simulink model "dspace"  (R2021b)
settings: Solver=FixedStepDiscrete  StartTime=0.0  StopTime=Inf  FixedStep=1e-3  RelTol=1e-3
PostLoadFcn:
  | , if any(exist('dsrtsu_mdlpostloadfcn', 'file') ~= 0), dsrtsu_mdlpostloadfcn('Execute', bdroot); end,
undefined symbols (not defined in the file): ami, amk1_setpoints_1, amk2_setpoints_1, amk3_setpoints_1, amk4_setpoints_1, as, digital, ebs, indicator, mcu_set_dbu_indicator_points, mcu_set_ecu_indicator_points, res_ntm_node_control
libraries: rtican x63, rti1401lib_dio_type3 x4, simulink x4, simulink_extras x1
(part 6 of 16)

== system dspace/CAN RX/amk1_actual_values_2 ==
  amk1_actual_values_21 : rtican/RTICAN Receive (RX)   Reserved1=[]  Reserved2=[]  Reserved3=[]  Reserved4=[]  SfcnMessage=[]  Msg_Struct=[]  BoardTypeNo=[]  BoardNo=[]  ChannelNo=[]  Parameters=[]  DialogFcn=[]  UnitName=[]  Revision=[]  UnitValues=[]  DSProperties=struct('RTI',struct('Version',uint32(5),'BlockType',struct('isSLSource',uint8(1),'isSLSink',uint8(1),'isHWSource',uint8(0),'isHWSink',uint8(0),'isSetup',uint8(0),'isInline',uint8(1),'isNonInline',uint8(0),'isInterrupt',uint8(0),'isChannelwise',uint8(0)),'IOBoardType','RTICAN','UnitType','MESSAGE','Identifier','RX','DialogType','MSVC','BlockSet','RTICAN','SlaveProcessor','CAN'))  RTIBlockInterface=struct('OutputPortsWidth',int32([1 1 1 1 1 1 1]),'OutputPortsActive',[1 1 1 1 1 1 1],'OutputPortsName',{{'amk1_temp_motor','amk1_temp_inverter','amk1_error_info','amk1_temp_igbt',['RX status'],['RX time'],['RX delta time']}},'OutputPortsDataType',{{'SS_DOUBLE','SS_DOUBLE','SS_DOUBLE','SS_DOUBLE','SS_DOUBLE','SS_DOUBLE','SS_DOUBLE'}},'OutputPortsLabel',{{'amk1_temp_motor','amk1_temp_inverter','amk1_error_info','amk1_temp_igbt','','',''}},'OutputPortsLabelMode','ON','InputPortsWidth',int32(0),'InputPortsActive',0,'DialogFcn','rtican_message_interface_gui','BlockDisplay',{{'','center'}},'IconTransparency','on','ParameterTunableNames',{{}},'InitLevel',3,'BlockName',struct('Token',{{'amk1_actual_values_2'}}),'SampleTime',{{-1}},'TriggerPort',{{'none'}},'EnablePort',{{'none'}})  RTIBlockParameters=struct('BoardTypeNo',{{1,'OFF',[]}},'BoardNo',{{1,'ON',[1 16]}},'ChannelNo',{{1,'ON',[1 2]}},'Parameters',{{struct('DataFileSupport',struct('DataFileSelectedMaster',1,'DataFileSelectedLocal',1,'DataFileName','c:\users\oscar\documents\github\sw_infrastructure\kthfspe_python\databases\can2.dbc|','DataFileDate',{{{['10-Jul-2022 04:24:51']}}},'SelectedFile','c:\users\oscar\documents\github\sw_infrastructure\kthfspe_python\databases\can2.dbc'),'Options',struct('StatusSelected',1,'TimeSelected',1,'DeltaTimeSelected',1,'BytePortSelected',0,'MessageLengthSelected',0,'TriggerPort',struct('Selected',0,'TriggerType',0),'UserCoding',struct('Selected',0,'InterfaceFile','UserDecodingFile','FcnName','UserDecodeFcn','InportSelected',0,'InportWidth',1,'OutportSelected',0,'OutportWidth',1),'EnablePortSelected',0,'SignalOnPortnameSelected',1,'UseRXService',0),'Message',struct('MsgOnBlocknameSelected',1,'MsgName','amk1_actual_values_2','MsgIdFormat',0,'MsgId',645,'MsgLength',8,'NumSignals',4,'SampleTime',-1,'Signal',struct('SgnName',{'amk1_temp_motor','amk1_temp_inverter','amk1_error_info','amk1_temp_igbt'},'SgnStartBit',{0,16,32,48},'SgnLength',{16,16,16,16},'SgnType',{0,0,0,0},'ModeValue',{-1,-1,-1,-1},'DataType',{1,1,0,1},'ByteLayout',{0,0,0,0},'Factor',{0.1,0.1,1,0.1},'Offset',{0,0,0,0},'SgnComment',{{['Motor temperature.']},{['Cold plate temperature.']},{['Diagnostic number.']},{['IGBT temperature.']}},'SgnUnit',{'C','C','','C'},'Min',{0,0,0,0},'Max',{0,0,0,0},'SLDataType',{'SS_DOUBLE','SS_DOUBLE','SS_DOUBLE','SS_DOUBLE'}),'MsgIdNumFormat',0,'MsgComment',{{['Periodic 5ms.']}}),'Version',1.2,'general',struct('isFromLib',0)),'OFF',[]}},'GroupId',{{struct('Group',{{'RTICAN'}},'No',2,'Behavior',{{'NAMECHANGE'}},'BlockType',{{'SINK'}},'NameChangeFlag',0),'OFF',[]}},'SFcnRTICANMessage',{{struct('MsgType','RX','SFcnPortType','Scalar','MsgName','amk1_actual_values_2','MsgIdFormat','STD','MsgId',645,'MsgLength',8,'NumSignals',4,'SampleTime',-1,'Signal',struct('SgnName',{'amk1_temp_motor','amk1_temp_inverter','amk1_error_info','amk1_temp_igbt'},'SgnStartBit',{0,16,32,48},'SgnLength',{16,16,16,16},'SgnType',{'standard','standard','standard','standard'},'ModeValue',{-1,-1,-1,-1},'DataType',{['signed int'],['signed int'],['unsigned int'],['signed int']},'ByteLayout',{['little endian'],['little endian'],['little endian'],['little endian']},'Factor',{0.1,0.1,1,0.1},'Offset',{0,0,0,0},'SLDataType',{'SS_DOUBLE','SS_DOUBLE','SS_DOUBLE','SS_DOUBLE'}),'StatusSelected','yes','TimeSelected','yes','DeltaTimeSelected','yes','BytePortSelected','no','MessageLengthSelected','no','TriggerPort',struct('Selected','no','TriggerType',0),'UserCoding',struct('Selected','no','InterfaceFile','UserDecodingFile','FcnName','UserDecodeFcn','InportSelected','no','InportWidth',1,'OutportSelected','no','OutportWidth',1),'EnablePortSelected','no','UseRXService','no','BoardType','DS1','BoardNo',1,'ControllerNo',2),'OFF',[]}},'TLCFileName',{{'rtican_rx_message','OFF',[]}})  RTISFcnParameters=struct('SFcnRTICANMessage','struct','TLCFileName','char')  RTIBlockParaDefault=struct('BoardTypeNo',4302,'BoardNo',1,'ChannelNo',1,'Parameters',struct('DataFileSupport',struct('DataFileSelectedMaster',0,'DataFileSelectedLocal',0,'DataFileName','','DataFileDate','','SelectedFile',['<no file selected>']),'Options',struct('StatusSelected',1,'TimeSelected',1,'DeltaTimeSelected',1,'BytePortSelected',0,'MessageLengthSelected',0,'TriggerPort',struct('Selected',0,'TriggerType','rising'),'UserCoding',struct('Selected',0,'InterfaceFile','UserDecodingFile','FcnName','UserDecodeFcn','InportSelected',0,'InportWidth',1,'OutportSelected',0,'OutportWidth',1),'EnablePortSelected',0,'SignalOnPortnameSelected',1,'UseRXService',0),'Message',struct('MsgOnBlocknameSelected',0,'MsgName',['RX Message'],'MsgIdFormat',0,'MsgId',100,'MsgLength',8,'NumSignals',1,'SampleTime',-1,'Signal',struct('SgnName',['RX signal'],'SgnStartBit',0,'SgnLength',8,'SgnType',0,'ModeValue',-1,'DataType',0,'SLDataType','SS_DOUBLE','ByteLayout',0,'Factor',1,'Offset',0,'Min',0,'Max',255,'SgnComment',{{}},'SgnUnit',''),'MsgIdNumFormat',0,'MsgComment',{{''}}),'Version',1.2,'general',struct('isFromLib',1)),'GroupId',struct('Group',{{'RTICAN'}},'No',1,'Behavior',{{'NAMECHANGE'}},'BlockType',{{'SINK'}},'NameChangeFlag',0),'SFcnRTICANMessage',struct('MsgType','RX','MsgName',['RX Message'],'MsgIdFormat','STD','MsgId',100,'MsgLength',8,'NumSignals',1,'SampleTime',-1,'Signal',struct('SgnName',['RX signal'],'SgnStartBit',0,'SgnLength',8,'SgnType','standard','ModeValue',-1,'DataType',['unsigned int'],'ByteLayout',['little endian'],'SLDataType','SS_DOUBLE','Factor',1,'Offset',0),'StatusSelected','yes','TimeSelected','yes','DeltaTimeSelected','yes','BytePortSelected','no','MessageLengthSelected','no','EnablePortSelected','no','UserCoding',struct('Selected','no','InterfaceFile','UserDecodingFile','FcnName','UserDecodeFcn','InportSelected','no','InportWidth',1,'OutportSelected','no','OutportWidth',1),'TriggerPort',struct('Selected','no','TriggerType','rising'),'UseRXService','no','BoardType','DS4302','BoardNo',1,'ControllerNo',1,'SFcnPortType','Scalar'),'TLCFileName','rtican_rx_message')
      settings: AttributesFormatString=Group Id: RTICAN2\n  SourceProductName=dSPACE RTI CAN Blockset
  clock_time : Clock
  sub_time : Sum  Inputs=+-
  amk1_temp_motor_bus : Outport  PortName=signals  Element=amk1_temp_motor
  amk1_temp_inverter_bus : Outport  PortName=signals  Element=amk1_temp_inverter
  amk1_error_info_bus : Outport  PortName=signals  Element=amk1_error_info
  amk1_temp_igbt_bus : Outport  PortName=signals  Element=amk1_temp_igbt
  status : Outport  Port=2
  time : Outport  Port=3
  delta : Outport  Port=4
  wires:
  clock_time/1 -> sub_time/1
  sub_time/1 -> time/1
  amk1_actual_values_21/5 -> status/1
  amk1_actual_values_21/6 -> sub_time/2
  amk1_actual_values_21/7 -> delta/1
  amk1_actual_values_21/1 -> amk1_temp_motor_bus/1  "amk1_temp_motor"
  amk1_actual_values_21/2 -> amk1_temp_inverter_bus/1  "amk1_temp_inverter"
  amk1_actual_values_21/3 -> amk1_error_info_bus/1  "amk1_error_info"
  amk1_actual_values_21/4 -> amk1_temp_igbt_bus/1  "amk1_temp_igbt"

== system dspace/CAN RX/amk2_actual_values_1 ==
  amk2_actual_values_11 : rtican/RTICAN Receive (RX)   Reserved1=[]  Reserved2=[]  Reserved3=[]  Reserved4=[]  SfcnMessage=[]  Msg_Struct=[]  BoardTypeNo=[]  BoardNo=[]  ChannelNo=[]  Parameters=[]  DialogFcn=[]  UnitName=[]  Revision=[]  UnitValues=[]  DSProperties=struct('RTI',struct('Version',uint32(5),'BlockType',struct('isSLSource',uint8(1),'isSLSink',uint8(1),'isHWSource',uint8(0),'isHWSink',uint8(0),'isSetup',uint8(0),'isInline',uint8(1),'isNonInline',uint8(0),'isInterrupt',uint8(0),'isChannelwise',uint8(0)),'IOBoardType','RTICAN','UnitType','MESSAGE','Identifier','RX','DialogType','MSVC','BlockSet','RTICAN','SlaveProcessor','CAN'))  RTIBlockInterface=struct('OutputPortsWidth',int32([1 1 1 1 1 1 1 1 1 1 1 1 1 1]),'OutputPortsActive',ones(1,14),'OutputPortsName',{{'amk2_system_ready','amk2_error','amk2_warning','amk2_status_quit_dc_on','amk2_status_dc_on','amk2_status_quit_inverter_on','amk2_status_inverter_on','amk2_status_derating','amk2_actual_velocity','amk2_torque_current','amk2_magnetizing_current',['RX status'],['RX time'],['RX delta time']}},'OutputPortsDataType',{{'SS_DOUBLE','SS_DOUBLE','SS_DOUBLE','SS_DOUBLE','SS_DOUBLE','SS_DOUBLE','SS_DOUBLE','SS_DOUBLE','SS_DOUBLE','SS_DOUBLE','SS_DOUBLE','SS_DOUBLE','SS_DOUBLE','SS_DOUBLE'}},'OutputPortsLabel',{{'amk2_system_ready','amk2_error','amk2_warning','amk2_status_quit_dc_on','amk2_status_dc_on','amk2_status_quit_inverter_on','amk2_status_inverter_on','amk2_status_derating','amk2_actual_velocity','amk2_torque_current','amk2_magnetizing_current','','',''}},'OutputPortsLabelMode','ON','InputPortsWidth',int32(0),'InputPortsActive',0,'DialogFcn','rtican_message_interface_gui','BlockDisplay',{{'','center'}},'IconTransparency','on','ParameterTunableNames',{{}},'InitLevel',3,'BlockName',struct('Token',{{'amk2_actual_values_1'}}),'SampleTime',{{-1}},'TriggerPort',{{'none'}},'EnablePort',{{'none'}})  RTIBlockParameters=struct('BoardTypeNo',{{1,'OFF',[]}},'BoardNo',{{1,'ON',[1 16]}},'ChannelNo',{{1,'ON',[1 2]}},'Parameters',{{struct('DataFileSupport',struct('DataFileSelectedMaster',1,'DataFileSelectedLocal',1,'DataFileName','c:\users\oscar\documents\github\sw_infrastructure\kthfspe_python\databases\can2.dbc|','DataFileDate',{{{['10-Jul-2022 04:24:51']}}},'SelectedFile','c:\users\oscar\documents\github\sw_infrastructure\kthfspe_python\databases\can2.dbc'),'Options',struct('StatusSelected',1,'TimeSelected',1,'DeltaTimeSelected',1,'BytePortSelected',0,'MessageLengthSelected',0,'TriggerPort',struct('Selected',0,'TriggerType',0),'UserCoding',struct('Selected',0,'InterfaceFile','UserDecodingFile','FcnName','UserDecodeFcn','InportSelected',0,'InportWidth',1,'OutportSelected',0,'OutportWidth',1),'EnablePortSelected',0,'SignalOnPortnameSelected',1,'UseRXService',0),'Message',struct('MsgOnBlocknameSelected',1,'MsgName','amk2_actual_values_1','MsgIdFormat',0,'MsgId',644,'MsgLength',8,'NumSignals',11,'SampleTime',-1,'Signal',struct('SgnName',{'amk2_system_ready','amk2_error','amk2_warning','amk2_status_quit_dc_on','amk2_status_dc_on','amk2_status_quit_inverter_on','amk2_status_inverter_on','amk2_status_derating','amk2_actual_velocity','amk2_torque_current','amk2_magnetizing_current'},'SgnStartBit',{8,9,10,11,12,13,14,15,16,32,48},'SgnLength',{1,1,1,1,1,1,1,1,16,16,16},'SgnType',{0,0,0,0,0,0,0,0,0,0,0},'ModeValue',{-1,-1,-1,-1,-1,-1,-1,-1,-1,-1,-1},'DataType',{0,0,0,0,0,0,0,0,1,1,1},'ByteLayout',{0,0,0,0,0,0,0,0,0,0,0},'Factor',{1,1,1,1,1,1,1,1,1,1,1},'Offset',{0,0,0,0,0,0,0,0,0,0,0},'SgnComment',{{''},{''},{''},{''},{''},{''},{''},{''},{''},{''},{''}},'SgnUnit',{'','','','','','','','','rpm','',''},'Min',{0,0,0,0,0,0,0,0,0,0,0},'Max',{0,0,0,0,0,0,0,0,0,0,0},'SLDataType',{'SS_DOUBLE','SS_DOUBLE','SS_DOUBLE','SS_DOUBLE','SS_DOUBLE','SS_DOUBLE','SS_DOUBLE','SS_DOUBLE','SS_DOUBLE','SS_DOUBLE','SS_DOUBLE'}),'MsgIdNumFormat',0,'MsgComment',{{['Periodic 5ms.']}}),'Version',1.2,'general',struct('isFromLib',0)),'OFF',[]}},'GroupId',{{struct('Group',{{'RTICAN'}},'No',2,'Behavior',{{'NAMECHANGE'}},'BlockType',{{'SINK'}},'NameChangeFlag',0),'OFF',[]}},'SFcnRTICANMessage',{{struct('MsgType','RX','SFcnPortType','Scalar','MsgName','amk2_actual_values_1','MsgIdFormat','STD','MsgId',644,'MsgLength',8,'NumSignals',11,'SampleTime',-1,'Signal',struct('SgnName',{'amk2_system_ready','amk2_error','amk2_warning','amk2_status_quit_dc_on','amk2_status_dc_on','amk2_status_quit_inverter_on','amk2_status_inverter_on','amk2_status_derating','amk2_actual_velocity','amk2_torque_current','amk2_magnetizing_current'},'SgnStartBit',{8,9,10,11,12,13,14,15,16,32,48},'SgnLength',{1,1,1,1,1,1,1,1,16,16,16},'SgnType',{'standard','standard','standard','standard','standard','standard','standard','standard','standard','standard','standard'},'ModeValue',{-1,-1,-1,-1,-1,-1,-1,-1,-1,-1,-1},'DataType',{['unsigned int'],['unsigned int'],['unsigned int'],['unsigned int'],['unsigned int'],['unsigned int'],['unsigned int'],['unsigned int'],['signed int'],['signed int'],['signed int']},'ByteLayout',{['little endian'],['little endian'],['little endian'],['little endian'],['little endian'],['little endian'],['little endian'],['little endian'],['little endian'],['little endian'],['little endian']},'Factor',{1,1,1,1,1,1,1,1,1,1,1},'Offset',{0,0,0,0,0,0,0,0,0,0,0},'SLDataType',{'SS_DOUBLE','SS_DOUBLE','SS_DOUBLE','SS_DOUBLE','SS_DOUBLE','SS_DOUBLE','SS_DOUBLE','SS_DOUBLE','SS_DOUBLE','SS_DOUBLE','SS_DOUBLE'}),'StatusSelected','yes','TimeSelected','yes','DeltaTimeSelected','yes','BytePortSelected','no','MessageLengthSelected','no','TriggerPort',struct('Selected','no','TriggerType',0),'UserCoding',struct('Selected','no','InterfaceFile','UserDecodingFile','FcnName','UserDecodeFcn','InportSelected','no','InportWidth',1,'OutportSelected','no','OutportWidth',1),'EnablePortSelected','no','UseRXService','no','BoardType','DS1','BoardNo',1,'ControllerNo',2),'OFF',[]}},'TLCFileName',{{'rtican_rx_message','OFF',[]}})  RTISFcnParameters=struct('SFcnRTICANMessage','struct','TLCFileName','char')  RTIBlockParaDefault=struct('BoardTypeNo',4302,'BoardNo',1,'ChannelNo',1,'Parameters',struct('DataFileSupport',struct('DataFileSelectedMaster',0,'DataFileSelectedLocal',0,'DataFileName','','DataFileDate','','SelectedFile',['<no file selected>']),'Options',struct('StatusSelected',1,'TimeSelected',1,'DeltaTimeSelected',1,'BytePortSelected',0,'MessageLengthSelected',0,'TriggerPort',struct('Selected',0,'TriggerType','rising'),'UserCoding',struct('Selected',0,'InterfaceFile','UserDecodingFile','FcnName','UserDecodeFcn','InportSelected',0,'InportWidth',1,'OutportSelected',0,'OutportWidth',1),'EnablePortSelected',0,'SignalOnPortnameSelected',1,'UseRXService',0),'Message',struct('MsgOnBlocknameSelected',0,'MsgName',['RX Message'],'MsgIdFormat',0,'MsgId',100,'MsgLength',8,'NumSignals',1,'SampleTime',-1,'Signal',struct('SgnName',['RX signal'],'SgnStartBit',0,'SgnLength',8,'SgnType',0,'ModeValue',-1,'DataType',0,'SLDataType','SS_DOUBLE','ByteLayout',0,'Factor',1,'Offset',0,'Min',0,'Max',255,'SgnComment',{{}},'SgnUnit',''),'MsgIdNumFormat',0,'MsgComment',{{''}}),'Version',1.2,'general',struct('isFromLib',1)),'GroupId',struct('Group',{{'RTICAN'}},'No',1,'Behavior',{{'NAMECHANGE'}},'BlockType',{{'SINK'}},'NameChangeFlag',0),'SFcnRTICANMessage',struct('MsgType','RX','MsgName',['RX Message'],'MsgIdFormat','STD','MsgId',100,'MsgLength',8,'NumSignals',1,'SampleTime',-1,'Signal',struct('SgnName',['RX signal'],'SgnStartBit',0,'SgnLength',8,'SgnType','standard','ModeValue',-1,'DataType',['unsigned int'],'ByteLayout',['little endian'],'SLDataType','SS_DOUBLE','Factor',1,'Offset',0),'StatusSelected','yes','TimeSelected','yes','DeltaTimeSelected','yes','BytePortSelected','no','MessageLengthSelected','no','EnablePortSelected','no','UserCoding',struct('Selected','no','InterfaceFile','UserDecodingFile','FcnName','UserDecodeFcn','InportSelected','no','InportWidth',1,'OutportSelected','no','OutportWidth',1),'TriggerPort',struct('Selected','no','TriggerType','rising'),'UseRXService','no','BoardType','DS4302','BoardNo',1,'ControllerNo',1,'SFcnPortType','Scalar'),'TLCFileName','rtican_rx_message')
      settings: AttributesFormatString=Group Id: RTICAN2\n  SourceProductName=dSPACE RTI CAN Blockset
  clock_time : Clock
  sub_time : Sum  Inputs=+-
  amk2_system_ready_bus : Outport  PortName=signals  Element=amk2_system_ready
  amk2_error_bus : Outport  PortName=signals  Element=amk2_error
  amk2_warning_bus : Outport  PortName=signals  Element=amk2_warning
  amk2_status_quit_dc_on_bus : Outport  PortName=signals  Element=amk2_status_quit_dc_on
  amk2_status_dc_on_bus : Outport  PortName=signals  Element=amk2_status_dc_on
  amk2_status_quit_inverter_on_bus : Outport  PortName=signals  Element=amk2_status_quit_inverter_on
  amk2_status_inverter_on_bus : Outport  PortName=signals  Element=amk2_status_inverter_on
  amk2_status_derating_bus : Outport  PortName=signals  Element=amk2_status_derating
  amk2_actual_velocity_bus : Outport  PortName=signals  Element=amk2_actual_velocity
  amk2_torque_current_bus : Outport  PortName=signals  Element=amk2_torque_current
  amk2_magnetizing_current_bus : Outport  PortName=signals  Element=amk2_magnetizing_current
  status : Outport  Port=2
  time : Outport  Port=3
  delta : Outport  Port=4
  wires:
  clock_time/1 -> sub_time/1
  sub_time/1 -> time/1
  amk2_actual_values_11/12 -> status/1
  amk2_actual_values_11/13 -> sub_time/2
  amk2_actual_values_11/14 -> delta/1
  amk2_actual_values_11/1 -> amk2_system_ready_bus/1  "amk2_system_ready"
  amk2_actual_values_11/2 -> amk2_error_bus/1  "amk2_error"
  amk2_actual_values_11/3 -> amk2_warning_bus/1  "amk2_warning"
  amk2_actual_values_11/4 -> amk2_status_quit_dc_on_bus/1  "amk2_status_quit_dc_on"
  amk2_actual_values_11/5 -> amk2_status_dc_on_bus/1  "amk2_status_dc_on"
  amk2_actual_values_11/6 -> amk2_status_quit_inverter_on_bus/1  "amk2_status_quit_inverter_on"
  amk2_actual_values_11/7 -> amk2_status_inverter_on_bus/1  "amk2_status_inverter_on"
  amk2_actual_values_11/8 -> amk2_status_derating_bus/1  "amk2_status_derating"
  amk2_actual_values_11/9 -> amk2_actual_velocity_bus/1  "amk2_actual_velocity"
  amk2_actual_values_11/10 -> amk2_torque_current_bus/1  "amk2_torque_current"
  amk2_actual_values_11/11 -> amk2_magnetizing_current_bus/1  "amk2_magnetizing_current"

== system dspace/CAN RX/amk2_actual_values_2 ==
  amk2_actual_values_21 : rtican/RTICAN Receive (RX)   Reserved1=[]  Reserved2=[]  Reserved3=[]  Reserved4=[]  SfcnMessage=[]  Msg_Struct=[]  BoardTypeNo=[]  BoardNo=[]  ChannelNo=[]  Parameters=[]  DialogFcn=[]  UnitName=[]  Revision=[]  UnitValues=[]  DSProperties=struct('RTI',struct('Version',uint32(5),'BlockType',struct('isSLSource',uint8(1),'isSLSink',uint8(1),'isHWSource',uint8(0),'isHWSink',uint8(0),'isSetup',uint8(0),'isInline',uint8(1),'isNonInline',uint8(0),'isInterrupt',uint8(0),'isChannelwise',uint8(0)),'IOBoardType','RTICAN','UnitType','MESSAGE','Identifier','RX','DialogType','MSVC','BlockSet','RTICAN','SlaveProcessor','CAN'))  RTIBlockInterface=struct('OutputPortsWidth',int32([1 1 1 1 1 1 1]),'OutputPortsActive',[1 1 1 1 1 1 1],'OutputPortsName',{{'amk2_temp_motor','amk2_temp_inverter','amk2_error_info','amk2_temp_igbt',['RX status'],['RX time'],['RX delta time']}},'OutputPortsDataType',{{'SS_DOUBLE','SS_DOUBLE','SS_DOUBLE','SS_DOUBLE','SS_DOUBLE','SS_DOUBLE','SS_DOUBLE'}},'OutputPortsLabel',{{'amk2_temp_motor','amk2_temp_inverter','amk2_error_info','amk2_temp_igbt','','',''}},'OutputPortsLabelMode','ON','InputPortsWidth',int32(0),'InputPortsActive',0,'DialogFcn','rtican_message_interface_gui','BlockDisplay',{{'','center'}},'IconTransparency','on','ParameterTunableNames',{{}},'InitLevel',3,'BlockName',struct('Token',{{'amk2_actual_values_2'}}),'SampleTime',{{-1}},'TriggerPort',{{'none'}},'EnablePort',{{'none'}})  RTIBlockParameters=struct('BoardTypeNo',{{1,'OFF',[]}},'BoardNo',{{1,'ON',[1 16]}},'ChannelNo',{{1,'ON',[1 2]}},'Parameters',{{struct('DataFileSupport',struct('DataFileSelectedMaster',1,'DataFileSelectedLocal',1,'DataFileName','c:\users\oscar\documents\github\sw_infrastructure\kthfspe_python\databases\can2.dbc|','DataFileDate',{{{['10-Jul-2022 04:24:51']}}},'SelectedFile','c:\users\oscar\documents\github\sw_infrastructure\kthfspe_python\databases\can2.dbc'),'Options',struct('StatusSelected',1,'TimeSelected',1,'DeltaTimeSelected',1,'BytePortSelected',0,'MessageLengthSelected',0,'TriggerPort',struct('Selected',0,'TriggerType',0),'UserCoding',struct('Selected',0,'InterfaceFile','UserDecodingFile','FcnName','UserDecodeFcn','InportSelected',0,'InportWidth',1,'OutportSelected',0,'OutportWidth',1),'EnablePortSelected',0,'SignalOnPortnameSelected',1,'UseRXService',0),'Message',struct('MsgOnBlocknameSelected',1,'MsgName','amk2_actual_values_2','MsgIdFormat',0,'MsgId',646,'MsgLength',8,'NumSignals',4,'SampleTime',-1,'Signal',struct('SgnName',{'amk2_temp_motor','amk2_temp_inverter','amk2_error_info','amk2_temp_igbt'},'SgnStartBit',{0,16,32,48},'SgnLength',{16,16,16,16},'SgnType',{0,0,0,0},'ModeValue',{-1,-1,-1,-1},'DataType',{1,1,0,1},'ByteLayout',{0,0,0,0},'Factor',{0.1,0.1,1,0.1},'Offset',{0,0,0,0},'SgnComment',{{''},{''},{''},{''}},'SgnUnit',{'C','C','','C'},'Min',{0,0,0,0},'Max',{0,0,0,0},'SLDataType',{'SS_DOUBLE','SS_DOUBLE','SS_DOUBLE','SS_DOUBLE'}),'MsgIdNumFormat',0,'MsgComment',{{['Periodic 5ms.']}}),'Version',1.2,'general',struct('isFromLib',0)),'OFF',[]}},'GroupId',{{struct('Group',{{'RTICAN'}},'No',2,'Behavior',{{'NAMECHANGE'}},'BlockType',{{'SINK'}},'NameChangeFlag',0),'OFF',[]}},'SFcnRTICANMessage',{{struct('MsgType','RX','SFcnPortType','Scalar','MsgName','amk2_actual_values_2','MsgIdFormat','STD','MsgId',646,'MsgLength',8,'NumSignals',4,'SampleTime',-1,'Signal',struct('SgnName',{'amk2_temp_motor','amk2_temp_inverter','amk2_error_info','amk2_temp_igbt'},'SgnStartBit',{0,16,32,48},'SgnLength',{16,16,16,16},'SgnType',{'standard','standard','standard','standard'},'ModeValue',{-1,-1,-1,-1},'DataType',{['signed int'],['signed int'],['unsigned int'],['signed int']},'ByteLayout',{['little endian'],['little endian'],['little endian'],['little endian']},'Factor',{0.1,0.1,1,0.1},'Offset',{0,0,0,0},'SLDataType',{'SS_DOUBLE','SS_DOUBLE','SS_DOUBLE','SS_DOUBLE'}),'StatusSelected','yes','TimeSelected','yes','DeltaTimeSelected','yes','BytePortSelected','no','MessageLengthSelected','no','TriggerPort',struct('Selected','no','TriggerType',0),'UserCoding',struct('Selected','no','InterfaceFile','UserDecodingFile','FcnName','UserDecodeFcn','InportSelected','no','InportWidth',1,'OutportSelected','no','OutportWidth',1),'EnablePortSelected','no','UseRXService','no','BoardType','DS1','BoardNo',1,'ControllerNo',2),'OFF',[]}},'TLCFileName',{{'rtican_rx_message','OFF',[]}})  RTISFcnParameters=struct('SFcnRTICANMessage','struct','TLCFileName','char')  RTIBlockParaDefault=struct('BoardTypeNo',4302,'BoardNo',1,'ChannelNo',1,'Parameters',struct('DataFileSupport',struct('DataFileSelectedMaster',0,'DataFileSelectedLocal',0,'DataFileName','','DataFileDate','','SelectedFile',['<no file selected>']),'Options',struct('StatusSelected',1,'TimeSelected',1,'DeltaTimeSelected',1,'BytePortSelected',0,'MessageLengthSelected',0,'TriggerPort',struct('Selected',0,'TriggerType','rising'),'UserCoding',struct('Selected',0,'InterfaceFile','UserDecodingFile','FcnName','UserDecodeFcn','InportSelected',0,'InportWidth',1,'OutportSelected',0,'OutportWidth',1),'EnablePortSelected',0,'SignalOnPortnameSelected',1,'UseRXService',0),'Message',struct('MsgOnBlocknameSelected',0,'MsgName',['RX Message'],'MsgIdFormat',0,'MsgId',100,'MsgLength',8,'NumSignals',1,'SampleTime',-1,'Signal',struct('SgnName',['RX signal'],'SgnStartBit',0,'SgnLength',8,'SgnType',0,'ModeValue',-1,'DataType',0,'SLDataType','SS_DOUBLE','ByteLayout',0,'Factor',1,'Offset',0,'Min',0,'Max',255,'SgnComment',{{}},'SgnUnit',''),'MsgIdNumFormat',0,'MsgComment',{{''}}),'Version',1.2,'general',struct('isFromLib',1)),'GroupId',struct('Group',{{'RTICAN'}},'No',1,'Behavior',{{'NAMECHANGE'}},'BlockType',{{'SINK'}},'NameChangeFlag',0),'SFcnRTICANMessage',struct('MsgType','RX','MsgName',['RX Message'],'MsgIdFormat','STD','MsgId',100,'MsgLength',8,'NumSignals',1,'SampleTime',-1,'Signal',struct('SgnName',['RX signal'],'SgnStartBit',0,'SgnLength',8,'SgnType','standard','ModeValue',-1,'DataType',['unsigned int'],'ByteLayout',['little endian'],'SLDataType','SS_DOUBLE','Factor',1,'Offset',0),'StatusSelected','yes','TimeSelected','yes','DeltaTimeSelected','yes','BytePortSelected','no','MessageLengthSelected','no','EnablePortSelected','no','UserCoding',struct('Selected','no','InterfaceFile','UserDecodingFile','FcnName','UserDecodeFcn','InportSelected','no','InportWidth',1,'OutportSelected','no','OutportWidth',1),'TriggerPort',struct('Selected','no','TriggerType','rising'),'UseRXService','no','BoardType','DS4302','BoardNo',1,'ControllerNo',1,'SFcnPortType','Scalar'),'TLCFileName','rtican_rx_message')
      settings: AttributesFormatString=Group Id: RTICAN2\n  SourceProductName=dSPACE RTI CAN Blockset
  clock_time : Clock
  sub_time : Sum  Inputs=+-
  amk2_temp_motor_bus : Outport  PortName=signals  Element=amk2_temp_motor
  amk2_temp_inverter_bus : Outport  PortName=signals  Element=amk2_temp_inverter
  amk2_error_info_bus : Outport  PortName=signals  Element=amk2_error_info
  amk2_temp_igbt_bus : Outport  PortName=signals  Element=amk2_temp_igbt
  status : Outport  Port=2
  time : Outport  Port=3
  delta : Outport  Port=4
  wires:
  clock_time/1 -> sub_time/1
  sub_time/1 -> time/1
  amk2_actual_values_21/5 -> status/1
  amk2_actual_values_21/6 -> sub_time/2
  amk2_actual_values_21/7 -> delta/1
  amk2_actual_values_21/1 -> amk2_temp_motor_bus/1  "amk2_temp_motor"
  amk2_actual_values_21/2 -> amk2_temp_inverter_bus/1  "amk2_temp_inverter"
  amk2_actual_values_21/3 -> amk2_error_info_bus/1  "amk2_error_info"
  amk2_actual_values_21/4 -> amk2_temp_igbt_bus/1  "amk2_temp_igbt"

== system dspace/CAN RX/amk3_actual_values_1 ==
  amk3_actual_values_11 : rtican/RTICAN Receive (RX)   Reserved1=[]  Reserved2=[]  Reserved3=[]  Reserved4=[]  SfcnMessage=[]  Msg_Struct=[]  BoardTypeNo=[]  BoardNo=[]  ChannelNo=[]  Parameters=[]  DialogFcn=[]  UnitName=[]  Revision=[]  UnitValues=[]  DSProperties=struct('RTI',struct('Version',uint32(5),'BlockType',struct('isSLSource',uint8(1),'isSLSink',uint8(1),'isHWSource',uint8(0),'isHWSink',uint8(0),'isSetup',uint8(0),'isInline',uint8(1),'isNonInline',uint8(0),'isInterrupt',uint8(0),'isChannelwise',uint8(0)),'IOBoardType','RTICAN','UnitType','MESSAGE','Identifier','RX','DialogType','MSVC','BlockSet','RTICAN','SlaveProcessor','CAN'))  RTIBlockInterface=struct('OutputPortsWidth',int32([1 1 1 1 1 1 1 1 1 1 1 1 1 1]),'OutputPortsActive',ones(1,14),'OutputPortsName',{{'amk3_system_ready','amk3_error','amk3_warning','amk3_status_quit_dc_on','amk3_status_dc_on','amk3_status_quit_inverter_on','amk3_status_inverter_on','amk3_status_derating','amk3_actual_velocity','amk3_torque_current','amk3_magnetizing_current',['RX status'],['RX time'],['RX delta time']}},'OutputPortsDataType',{{'SS_DOUBLE','SS_DOUBLE','SS_DOUBLE','SS_DOUBLE','SS_DOUBLE','SS_DOUBLE','SS_DOUBLE','SS_DOUBLE','SS_DOUBLE','SS_DOUBLE','SS_DOUBLE','SS_DOUBLE','SS_DOUBLE','SS_DOUBLE'}},'OutputPortsLabel',{{'amk3_system_ready','amk3_error','amk3_warning','amk3_status_quit_dc_on','amk3_status_dc_on','amk3_status_quit_inverter_on','amk3_status_inverter_on','amk3_status_derating','amk3_actual_velocity','amk3_torque_current','amk3_magnetizing_current','','',''}},'OutputPortsLabelMode','ON','InputPortsWidth',int32(0),'InputPortsActive',0,'DialogFcn','rtican_message_interface_gui','BlockDisplay',{{'','center'}},'IconTransparency','on','ParameterTunableNames',{{}},'InitLevel',3,'BlockName',struct('Token',{{'amk3_actual_values_1'}}),'SampleTime',{{-1}},'TriggerPort',{{'none'}},'EnablePort',{{'none'}})  RTIBlockParameters=struct('BoardTypeNo',{{1,'OFF',[]}},'BoardNo',{{1,'ON',[1 16]}},'ChannelNo',{{1,'ON',[1 2]}},'Parameters',{{struct('DataFileSupport',struct('DataFileSelectedMaster',1,'DataFileSelectedLocal',1,'DataFileName','c:\users\oscar\documents\github\sw_infrastructure\kthfspe_python\databases\can2.dbc|','DataFileDate',{{{['10-Jul-2022 04:24:51']}}},'SelectedFile','c:\users\oscar\documents\github\sw_infrastructure\kthfspe_python\databases\can2.dbc'),'Options',struct('StatusSelected',1,'TimeSelected',1,'DeltaTimeSelected',1,'BytePortSelected',0,'MessageLengthSelected',0,'TriggerPort',struct('Selected',0,'TriggerType',0),'UserCoding',struct('Selected',0,'InterfaceFile','UserDecodingFile','FcnName','UserDecodeFcn','InportSelected',0,'InportWidth',1,'OutportSelected',0,'OutportWidth',1),'EnablePortSelected',0,'SignalOnPortnameSelected',1,'UseRXService',0),'Message',struct('MsgOnBlocknameSelected',1,'MsgName','amk3_actual_values_1','MsgIdFormat',0,'MsgId',647,'MsgLength',8,'NumSignals',11,'SampleTime',-1,'Signal',struct('SgnName',{'amk3_system_ready','amk3_error','amk3_warning','amk3_status_quit_dc_on','amk3_status_dc_on','amk3_status_quit_inverter_on','amk3_status_inverter_on','amk3_status_derating','amk3_actual_velocity','amk3_torque_current','amk3_magnetizing_current'},'SgnStartBit',{8,9,10,11,12,13,14,15,16,32,48},'SgnLength',{1,1,1,1,1,1,1,1,16,16,16},'SgnType',{0,0,0,0,0,0,0,0,0,0,0},'ModeValue',{-1,-1,-1,-1,-1,-1,-1,-1,-1,-1,-1},'DataType',{0,0,0,0,0,0,0,0,1,1,1},'ByteLayout',{0,0,0,0,0,0,0,0,0,0,0},'Factor',{1,1,1,1,1,1,1,1,1,1,1},'Offset',{0,0,0,0,0,0,0,0,0,0,0},'SgnComment',{{''},{''},{''},{''},{''},{''},{''},{''},{''},{''},{''}},'SgnUnit',{'','','','','','','','','rpm','',''},'Min',{0,0,0,0,0,0,0,0,0,0,0},'Max',{0,0,0,0,0,0,0,0,0,0,0},'SLDataType',{'SS_DOUBLE','SS_DOUBLE','SS_DOUBLE','SS_DOUBLE','SS_DOUBLE','SS_DOUBLE','SS_DOUBLE','SS_DOUBLE','SS_DOUBLE','SS_DOUBLE','SS_DOUBLE'}),'MsgIdNumFormat',0,'MsgComment',{{['Periodic 5ms.']}}),'Version',1.2,'general',struct('isFromLib',0)),'OFF',[]}},'GroupId',{{struct('Group',{{'RTICAN'}},'No',2,'Behavior',{{'NAMECHANGE'}},'BlockType',{{'SINK'}},'NameChangeFlag',0),'OFF',[]}},'SFcnRTICANMessage',{{struct('MsgType','RX','SFcnPortType','Scalar','MsgName','amk3_actual_values_1','MsgIdFormat','STD','MsgId',647,'MsgLength',8,'NumSignals',11,'SampleTime',-1,'Signal',struct('SgnName',{'amk3_system_ready','amk3_error','amk3_warning','amk3_status_quit_dc_on','amk3_status_dc_on','amk3_status_quit_inverter_on','amk3_status_inverter_on','amk3_status_derating','amk3_actual_velocity','amk3_torque_current','amk3_magnetizing_current'},'SgnStartBit',{8,9,10,11,12,13,14,15,16,32,48},'SgnLength',{1,1,1,1,1,1,1,1,16,16,16},'SgnType',{'standard','standard','standard','standard','standard','standard','standard','standard','standard','standard','standard'},'ModeValue',{-1,-1,-1,-1,-1,-1,-1,-1,-1,-1,-1},'DataType',{['unsigned int'],['unsigned int'],['unsigned int'],['unsigned int'],['unsigned int'],['unsigned int'],['unsigned int'],['unsigned int'],['signed int'],['signed int'],['signed int']},'ByteLayout',{['little endian'],['little endian'],['little endian'],['little endian'],['little endian'],['little endian'],['little endian'],['little endian'],['little endian'],['little endian'],['little endian']},'Factor',{1,1,1,1,1,1,1,1,1,1,1},'Offset',{0,0,0,0,0,0,0,0,0,0,0},'SLDataType',{'SS_DOUBLE','SS_DOUBLE','SS_DOUBLE','SS_DOUBLE','SS_DOUBLE','SS_DOUBLE','SS_DOUBLE','SS_DOUBLE','SS_DOUBLE','SS_DOUBLE','SS_DOUBLE'}),'StatusSelected','yes','TimeSelected','yes','DeltaTimeSelected','yes','BytePortSelected','no','MessageLengthSelected','no','TriggerPort',struct('Selected','no','TriggerType',0),'UserCoding',struct('Selected','no','InterfaceFile','UserDecodingFile','FcnName','UserDecodeFcn','InportSelected','no','InportWidth',1,'OutportSelected','no','OutportWidth',1),'EnablePortSelected','no','UseRXService','no','BoardType','DS1','BoardNo',1,'ControllerNo',2),'OFF',[]}},'TLCFileName',{{'rtican_rx_message','OFF',[]}})  RTISFcnParameters=struct('SFcnRTICANMessage','struct','TLCFileName','char')  RTIBlockParaDefault=struct('BoardTypeNo',4302,'BoardNo',1,'ChannelNo',1,'Parameters',struct('DataFileSupport',struct('DataFileSelectedMaster',0,'DataFileSelectedLocal',0,'DataFileName','','DataFileDate','','SelectedFile',['<no file selected>']),'Options',struct('StatusSelected',1,'TimeSelected',1,'DeltaTimeSelected',1,'BytePortSelected',0,'MessageLengthSelected',0,'TriggerPort',struct('Selected',0,'TriggerType','rising'),'UserCoding',struct('Selected',0,'InterfaceFile','UserDecodingFile','FcnName','UserDecodeFcn','InportSelected',0,'InportWidth',1,'OutportSelected',0,'OutportWidth',1),'EnablePortSelected',0,'SignalOnPortnameSelected',1,'UseRXService',0),'Message',struct('MsgOnBlocknameSelected',0,'MsgName',['RX Message'],'MsgIdFormat',0,'MsgId',100,'MsgLength',8,'NumSignals',1,'SampleTime',-1,'Signal',struct('SgnName',['RX signal'],'SgnStartBit',0,'SgnLength',8,'SgnType',0,'ModeValue',-1,'DataType',0,'SLDataType','SS_DOUBLE','ByteLayout',0,'Factor',1,'Offset',0,'Min',0,'Max',255,'SgnComment',{{}},'SgnUnit',''),'MsgIdNumFormat',0,'MsgComment',{{''}}),'Version',1.2,'general',struct('isFromLib',1)),'GroupId',struct('Group',{{'RTICAN'}},'No',1,'Behavior',{{'NAMECHANGE'}},'BlockType',{{'SINK'}},'NameChangeFlag',0),'SFcnRTICANMessage',struct('MsgType','RX','MsgName',['RX Message'],'MsgIdFormat','STD','MsgId',100,'MsgLength',8,'NumSignals',1,'SampleTime',-1,'Signal',struct('SgnName',['RX signal'],'SgnStartBit',0,'SgnLength',8,'SgnType','standard','ModeValue',-1,'DataType',['unsigned int'],'ByteLayout',['little endian'],'SLDataType','SS_DOUBLE','Factor',1,'Offset',0),'StatusSelected','yes','TimeSelected','yes','DeltaTimeSelected','yes','BytePortSelected','no','MessageLengthSelected','no','EnablePortSelected','no','UserCoding',struct('Selected','no','InterfaceFile','UserDecodingFile','FcnName','UserDecodeFcn','InportSelected','no','InportWidth',1,'OutportSelected','no','OutportWidth',1),'TriggerPort',struct('Selected','no','TriggerType','rising'),'UseRXService','no','BoardType','DS4302','BoardNo',1,'ControllerNo',1,'SFcnPortType','Scalar'),'TLCFileName','rtican_rx_message')
      settings: AttributesFormatString=Group Id: RTICAN2\n  SourceProductName=dSPACE RTI CAN Blockset
  clock_time : Clock
  sub_time : Sum  Inputs=+-
  amk3_system_ready_bus : Outport  PortName=signals  Element=amk3_system_ready
  amk3_error_bus : Outport  PortName=signals  Element=amk3_error
  amk3_warning_bus : Outport  PortName=signals  Element=amk3_warning
  amk3_status_quit_dc_on_bus : Outport  PortName=signals  Element=amk3_status_quit_dc_on
  amk3_status_dc_on_bus : Outport  PortName=signals  Element=amk3_status_dc_on
  amk3_status_quit_inverter_on_bus : Outport  PortName=signals  Element=amk3_status_quit_inverter_on
  amk3_status_inverter_on_bus : Outport  PortName=signals  Element=amk3_status_inverter_on
  amk3_status_derating_bus : Outport  PortName=signals  Element=amk3_status_derating
  amk3_actual_velocity_bus : Outport  PortName=signals  Element=amk3_actual_velocity
  amk3_torque_current_bus : Outport  PortName=signals  Element=amk3_torque_current
  amk3_magnetizing_current_bus : Outport  PortName=signals  Element=amk3_magnetizing_current
  status : Outport  Port=2
  time : Outport  Port=3
  delta : Outport  Port=4
  wires:
  clock_time/1 -> sub_time/1
  sub_time/1 -> time/1
  amk3_actual_values_11/12 -> status/1
  amk3_actual_values_11/13 -> sub_time/2
  amk3_actual_values_11/14 -> delta/1
  amk3_actual_values_11/1 -> amk3_system_ready_bus/1  "amk3_system_ready"
  amk3_actual_values_11/2 -> amk3_error_bus/1  "amk3_error"
  amk3_actual_values_11/3 -> amk3_warning_bus/1  "amk3_warning"
  amk3_actual_values_11/4 -> amk3_status_quit_dc_on_bus/1  "amk3_status_quit_dc_on"
  amk3_actual_values_11/5 -> amk3_status_dc_on_bus/1  "amk3_status_dc_on"
  amk3_actual_values_11/6 -> amk3_status_quit_inverter_on_bus/1  "amk3_status_quit_inverter_on"
  amk3_actual_values_11/7 -> amk3_status_inverter_on_bus/1  "amk3_status_inverter_on"
  amk3_actual_values_11/8 -> amk3_status_derating_bus/1  "amk3_status_derating"
  amk3_actual_values_11/9 -> amk3_actual_velocity_bus/1  "amk3_actual_velocity"
  amk3_actual_values_11/10 -> amk3_torque_current_bus/1  "amk3_torque_current"
  amk3_actual_values_11/11 -> amk3_magnetizing_current_bus/1  "amk3_magnetizing_current"

== system dspace/CAN RX/amk3_actual_values_2 ==
  amk3_actual_values_21 : rtican/RTICAN Receive (RX)   Reserved1=[]  Reserved2=[]  Reserved3=[]  Reserved4=[]  SfcnMessage=[]  Msg_Struct=[]  BoardTypeNo=[]  BoardNo=[]  ChannelNo=[]  Parameters=[]  DialogFcn=[]  UnitName=[]  Revision=[]  UnitValues=[]  DSProperties=struct('RTI',struct('Version',uint32(5),'BlockType',struct('isSLSource',uint8(1),'isSLSink',uint8(1),'isHWSource',uint8(0),'isHWSink',uint8(0),'isSetup',uint8(0),'isInline',uint8(1),'isNonInline',uint8(0),'isInterrupt',uint8(0),'isChannelwise',uint8(0)),'IOBoardType','RTICAN','UnitType','MESSAGE','Identifier','RX','DialogType','MSVC','BlockSet','RTICAN','SlaveProcessor','CAN'))  RTIBlockInterface=struct('OutputPortsWidth',int32([1 1 1 1 1 1 1]),'OutputPortsActive',[1 1 1 1 1 1 1],'OutputPortsName',{{'amk3_temp_motor','amk3_temp_inverter','amk3_error_info','amk3_temp_igbt',['RX status'],['RX time'],['RX delta time']}},'OutputPortsDataType',{{'SS_DOUBLE','SS_DOUBLE','SS_DOUBLE','SS_DOUBLE','SS_DOUBLE','SS_DOUBLE','SS_DOUBLE'}},'OutputPortsLabel',{{'amk3_temp_motor','amk3_temp_inverter','amk3_error_info','amk3_temp_igbt','','',''}},'OutputPortsLabelMode','ON','InputPortsWidth',int32(0),'InputPortsActive',0,'DialogFcn','rtican_message_interface_gui','BlockDisplay',{{'','center'}},'IconTransparency','on','ParameterTunableNames',{{}},'InitLevel',3,'BlockName',struct('Token',{{'amk3_actual_values_2'}}),'SampleTime',{{-1}},'TriggerPort',{{'none'}},'EnablePort',{{'none'}})  RTIBlockParameters=struct('BoardTypeNo',{{1,'OFF',[]}},'BoardNo',{{1,'ON',[1 16]}},'ChannelNo',{{1,'ON',[1 2]}},'Parameters',{{struct('DataFileSupport',struct('DataFileSelectedMaster',1,'DataFileSelectedLocal',1,'DataFileName','c:\users\oscar\documents\github\sw_infrastructure\kthfspe_python\databases\can2.dbc|','DataFileDate',{{{['10-Jul-2022 04:24:51']}}},'SelectedFile','c:\users\oscar\documents\github\sw_infrastructure\kthfspe_python\databases\can2.dbc'),'Options',struct('StatusSelected',1,'TimeSelected',1,'DeltaTimeSelected',1,'BytePortSelected',0,'MessageLengthSelected',0,'TriggerPort',struct('Selected',0,'TriggerType',0),'UserCoding',struct('Selected',0,'InterfaceFile','UserDecodingFile','FcnName','UserDecodeFcn','InportSelected',0,'InportWidth',1,'OutportSelected',0,'OutportWidth',1),'EnablePortSelected',0,'SignalOnPortnameSelected',1,'UseRXService',0),'Message',struct('MsgOnBlocknameSelected',1,'MsgName','amk3_actual_values_2','MsgIdFormat',0,'MsgId',649,'MsgLength',8,'NumSignals',4,'SampleTime',-1,'Signal',struct('SgnName',{'amk3_temp_motor','amk3_temp_inverter','amk3_error_info','amk3_temp_igbt'},'SgnStartBit',{0,16,32,48},'SgnLength',{16,16,16,16},'SgnType',{0,0,0,0},'ModeValue',{-1,-1,-1,-1},'DataType',{1,1,0,1},'ByteLayout',{0,0,0,0},'Factor',{0.1,0.1,1,0.1},'Offset',{0,0,0,0},'SgnComment',{{''},{''},{''},{''}},'SgnUnit',{'C','C','','C'},'Min',{0,0,0,0},'Max',{0,0,0,0},'SLDataType',{'SS_DOUBLE','SS_DOUBLE','SS_DOUBLE','SS_DOUBLE'}),'MsgIdNumFormat',0,'MsgComment',{{['Periodic 5ms.']}}),'Version',1.2,'general',struct('isFromLib',0)),'OFF',[]}},'GroupId',{{struct('Group',{{'RTICAN'}},'No',2,'Behavior',{{'NAMECHANGE'}},'BlockType',{{'SINK'}},'NameChangeFlag',0),'OFF',[]}},'SFcnRTICANMessage',{{struct('MsgType','RX','SFcnPortType','Scalar','MsgName','amk3_actual_values_2','MsgIdFormat','STD','MsgId',649,'MsgLength',8,'NumSignals',4,'SampleTime',-1,'Signal',struct('SgnName',{'amk3_temp_motor','amk3_temp_inverter','amk3_error_info','amk3_temp_igbt'},'SgnStartBit',{0,16,32,48},'SgnLength',{16,16,16,16},'SgnType',{'standard','standard','standard','standard'},'ModeValue',{-1,-1,-1,-1},'DataType',{['signed int'],['signed int'],['unsigned int'],['signed int']},'ByteLayout',{['little endian'],['little endian'],['little endian'],['little endian']},'Factor',{0.1,0.1,1,0.1},'Offset',{0,0,0,0},'SLDataType',{'SS_DOUBLE','SS_DOUBLE','SS_DOUBLE','SS_DOUBLE'}),'StatusSelected','yes','TimeSelected','yes','DeltaTimeSelected','yes','BytePortSelected','no','MessageLengthSelected','no','TriggerPort',struct('Selected','no','TriggerType',0),'UserCoding',struct('Selected','no','InterfaceFile','UserDecodingFile','FcnName','UserDecodeFcn','InportSelected','no','InportWidth',1,'OutportSelected','no','OutportWidth',1),'EnablePortSelected','no','UseRXService','no','BoardType','DS1','BoardNo',1,'ControllerNo',2),'OFF',[]}},'TLCFileName',{{'rtican_rx_message','OFF',[]}})  RTISFcnParameters=struct('SFcnRTICANMessage','struct','TLCFileName','char')  RTIBlockParaDefault=struct('BoardTypeNo',4302,'BoardNo',1,'ChannelNo',1,'Parameters',struct('DataFileSupport',struct('DataFileSelectedMaster',0,'DataFileSelectedLocal',0,'DataFileName','','DataFileDate','','SelectedFile',['<no file selected>']),'Options',struct('StatusSelected',1,'TimeSelected',1,'DeltaTimeSelected',1,'BytePortSelected',0,'MessageLengthSelected',0,'TriggerPort',struct('Selected',0,'TriggerType','rising'),'UserCoding',struct('Selected',0,'InterfaceFile','UserDecodingFile','FcnName','UserDecodeFcn','InportSelected',0,'InportWidth',1,'OutportSelected',0,'OutportWidth',1),'EnablePortSelected',0,'SignalOnPortnameSelected',1,'UseRXService',0),'Message',struct('MsgOnBlocknameSelected',0,'MsgName',['RX Message'],'MsgIdFormat',0,'MsgId',100,'MsgLength',8,'NumSignals',1,'SampleTime',-1,'Signal',struct('SgnName',['RX signal'],'SgnStartBit',0,'SgnLength',8,'SgnType',0,'ModeValue',-1,'DataType',0,'SLDataType','SS_DOUBLE','ByteLayout',0,'Factor',1,'Offset',0,'Min',0,'Max',255,'SgnComment',{{}},'SgnUnit',''),'MsgIdNumFormat',0,'MsgComment',{{''}}),'Version',1.2,'general',struct('isFromLib',1)),'GroupId',struct('Group',{{'RTICAN'}},'No',1,'Behavior',{{'NAMECHANGE'}},'BlockType',{{'SINK'}},'NameChangeFlag',0),'SFcnRTICANMessage',struct('MsgType','RX','MsgName',['RX Message'],'MsgIdFormat','STD','MsgId',100,'MsgLength',8,'NumSignals',1,'SampleTime',-1,'Signal',struct('SgnName',['RX signal'],'SgnStartBit',0,'SgnLength',8,'SgnType','standard','ModeValue',-1,'DataType',['unsigned int'],'ByteLayout',['little endian'],'SLDataType','SS_DOUBLE','Factor',1,'Offset',0),'StatusSelected','yes','TimeSelected','yes','DeltaTimeSelected','yes','BytePortSelected','no','MessageLengthSelected','no','EnablePortSelected','no','UserCoding',struct('Selected','no','InterfaceFile','UserDecodingFile','FcnName','UserDecodeFcn','InportSelected','no','InportWidth',1,'OutportSelected','no','OutportWidth',1),'TriggerPort',struct('Selected','no','TriggerType','rising'),'UseRXService','no','BoardType','DS4302','BoardNo',1,'ControllerNo',1,'SFcnPortType','Scalar'),'TLCFileName','rtican_rx_message')
      settings: AttributesFormatString=Group Id: RTICAN2\n  SourceProductName=dSPACE RTI CAN Blockset
  clock_time : Clock
  sub_time : Sum  Inputs=+-
  amk3_temp_motor_bus : Outport  PortName=signals  Element=amk3_temp_motor
  amk3_temp_inverter_bus : Outport  PortName=signals  Element=amk3_temp_inverter
  amk3_error_info_bus : Outport  PortName=signals  Element=amk3_error_info
  amk3_temp_igbt_bus : Outport  PortName=signals  Element=amk3_temp_igbt
  status : Outport  Port=2
  time : Outport  Port=3
  delta : Outport  Port=4
  wires:
  clock_time/1 -> sub_time/1
  sub_time/1 -> time/1
  amk3_actual_values_21/5 -> status/1
  amk3_actual_values_21/6 -> sub_time/2
  amk3_actual_values_21/7 -> delta/1
  amk3_actual_values_21/1 -> amk3_temp_motor_bus/1  "amk3_temp_motor"
  amk3_actual_values_21/2 -> amk3_temp_inverter_bus/1  "amk3_temp_inverter"
  amk3_actual_values_21/3 -> amk3_error_info_bus/1  "amk3_error_info"
  amk3_actual_values_21/4 -> amk3_temp_igbt_bus/1  "amk3_temp_igbt"
